simulink model "ibvs_lite_model"  (R2020b)
settings: Solver=ode45  StartTime=0.0  StopTime=inf  RelTol=1e-3  EnableMultiTasking=on
values from neighbouring files (symbols this model uses):
  q0 = zeros(7,1)    [setup.m]
  x0 = [T.t', tr2rpy(T)]    [setup.m]
undefined symbols (not defined in the file or in its folder): cond, LWR, mkgrid, nofriction, transl, troty, trotz
libraries: roblocks x19, simulink x4
(part 1 of 2)
settings Model: Creator=corkep  LastModifiedBy=kika
settings SolverCC: AlgebraicLoopSolver=LineSearch
settings DataIOCC: LimitDataPoints=on  SaveFormat=Array  TimeSaveName=t  OutputSaveName=y  ReturnWorkspaceOutputsName=opspace
settings OptimizationCC: LifeSpan=inf
settings DebuggingCC: AllowSymbolicDim=off  SFUnexpectedBacktrackingDiag=warning  SFNoUnconditionalDefaultTransitionDiag=warning  SFExecutionAtInitializationDiag=none  ArithmeticOperatorsInVariantConditions=warning
settings ModelReferenceCC: PropagateSignalLabelsOutOfModel=off
settings SFSimCC: SimUseLocalCustomCode=off  CustomCodeUndefinedFunction=UseInterfaceOnly
settings RTWCC: RTWUseLocalCustomCode=off
settings CodeAppCC: StateflowObjectComments=on
settings GRTTargetCC: TargetLangStandard=C89/C90 (ANSI)
settings ConfigComp: CovMetricSettings=dw  CovSaveCumulativeToWorkspaceVar=on  CovSaveSingleToWorkspaceVar=on  CovExternalEMLEnable=off

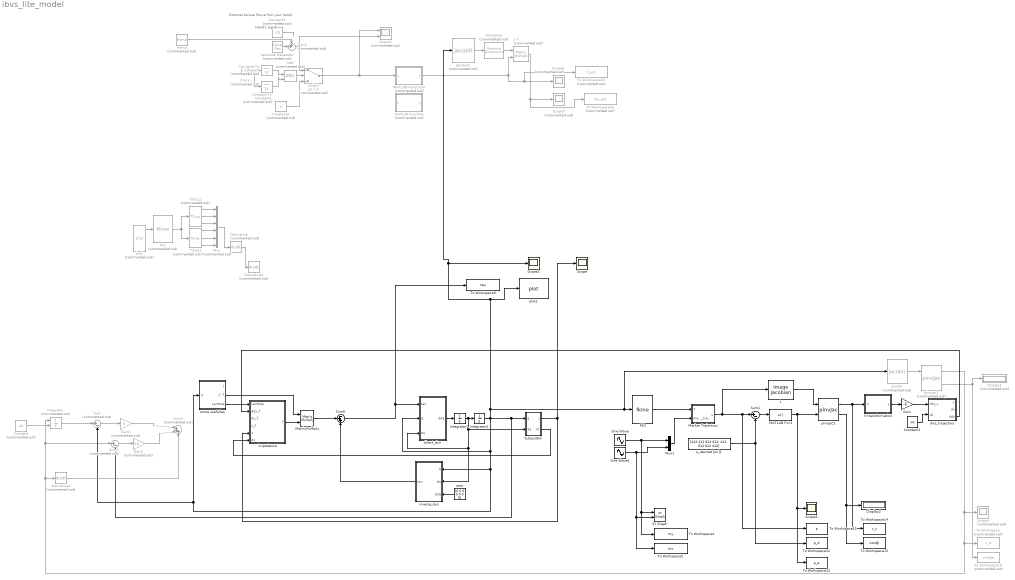
== system ibvs_lite_model ==
  note: Hand's signal
  note: External torque (force fron your hand)
  AND : Logic  Commented=on  IconShape=distinctive  AllPortsSameDT=off  OutDataTypeStr=boolean
  Clock : Clock  Commented=on
  Compare To Constant : simulink/Logic and Bit Operations/Compare To Constant  Commented=on  relop=>=  const=10  OutDataTypeStr=boolean
  Compare To Constant1 : simulink/Logic and Bit Operations/Compare To Constant  Commented=on  relop=<=  const=15  OutDataTypeStr=boolean
  Constant : Constant  Commented=on  Value=q0
  Constant1 : Constant  Value=x0
  Constant3 : Constant  Commented=on  Value=0
  Constant4 : Constant  Commented=on  Value=-25
  Derivative : Derivative  Commented=on
  Derivative1 : Derivative  Commented=on
  Derivative2 : Derivative  Commented=on
  Display1 : Display  Commented=on
  Display2 : Display
  FK1 : roblocks/Arm/fkine  Commented=on  robot=LWR
  FK2 : roblocks/Arm/fkine  robot=nofriction(LWR)
  Gain : Gain  Gain=-6
  Gain1 : Gain  Commented=on  Gain=5
  Gain2 : Gain  Commented=on  Gain=10
  Integrator : Integrator  Commented=on  InitialConditionSource=external  InitialCondition=q0'
  Integrator1 : Integrator
  Integrator2 : Integrator  InitialCondition=q0
  J' F : Product  Commented=on  Multiplication=Matrix(*)
  Jacobian : roblocks/Arm/jacob0   Commented=on  robot=LWR
  L : roblocks/Vision/image Jacobian  cam=cam  z=1
  MATLAB Fcn1 : MATLABFcn  MATLABFcn=u(:)  Output1D=off
  MATLAB Function : MATLAB Function  Commented=on  TreatAsAtomicUnit=on
  MATLAB Function3 : MATLAB Function  Commented=on  TreatAsAtomicUnit=on
  Marker Trajectory : Subsystem
  MatrixMultiply : Product  Multiplication=Matrix(*)
  Mux : Mux  Commented=on  Inputs=6
  Mux1 : Mux  Inputs=2
  Ramp : simulink/Sources/Ramp  Commented=on  slope=1  start=10  InitialOutput=-25
  Sawtooth Generator : SignalGenerator  Commented=on  Amplitude=18  Frequency=0.1  Units=rad/sec
  Scope : Scope
  Scope1 : Scope  Commented=on
  Scope2 : Scope
  Scope3 : Scope  Commented=on  NumInputPorts=2
  Scope4 : Scope
  Scope5 : Scope  Commented=on
  Scope6 : Scope  Commented=on
  Sine Wave : Sin  Amplitude=0.3  Frequency=0.3  SampleTime=0
  Sine Wave1 : Sin  Amplitude=0.3  Frequency=0.3  Phase=pi/2  SampleTime=0
  Subsystem : Subsystem
  Sum : Sum  Commented=on  Inputs=|+-
  Sum1 : Sum  Inputs=|+-
  Sum2 : Sum  Commented=on  Inputs=|+-
  Sum3 : Sum  Commented=on  Inputs=++|
  Sum4 : Sum  Commented=on  Inputs=|+++
  Sum6 : Sum  Inputs=-++  InputSameDT=on  SaturateOnIntegerOverflow=on  OutDataTypeStr=Inherit: Same as first input
  Switch : Switch  Commented=on  Criteria=u2 > Threshold
  T2rpy1 : roblocks/Toolbox/T2rpy  Commented=on  sequence=ZYX  degrees=off
  T2xyz1 : roblocks/Toolbox/T2xyz  Commented=on
  To Workspace : ToWorkspace  Commented=on  VariableName=v_e  SaveFormat=Timeseries  SampleTime=-1
  To Workspace10 : ToWorkspace  Commented=on  VariableName=f_ext  SaveFormat=Timeseries  SampleTime=-1
  To Workspace11 : ToWorkspace  VariableName=p  SaveFormat=Timeseries  SampleTime=-1
  To Workspace12 : ToWorkspace  VariableName=p_d  SaveFormat=Timeseries  SampleTime=-1
  To Workspace13 : ToWorkspace  VariableName=p_e  SaveFormat=Timeseries  SampleTime=-1
  To Workspace14 : ToWorkspace  VariableName=v_c  SaveFormat=Timeseries  SampleTime=-1
  To Workspace15 : ToWorkspace  VariableName=condJi  SaveFormat=Timeseries  SampleTime=-1
  To Workspace16 : ToWorkspace  Commented=on  VariableName=tau_ext  SaveFormat=Timeseries  SampleTime=-1
  To Workspace19 : ToWorkspace  Commented=on  VariableName=condJe  SaveFormat=Timeseries  SampleTime=-1
  To Workspace4 : ToWorkspace  VariableName=my  SaveFormat=Timeseries  SampleTime=-1
  To Workspace5 : ToWorkspace  VariableName=mz  SaveFormat=Timeseries  SampleTime=-1
  To Workspace9 : ToWorkspace  VariableName=tau  SaveFormat=Timeseries  SampleTime=-1
  V transformation : MATLAB Function  TreatAsAtomicUnit=on
  XY Graph : simulink/Sinks/XY Graph  xmin=-1  xmax=1  ymin=-1  ymax=1  st=-1
  "direct_dyn " : MATLAB Function  TreatAsAtomicUnit=on
  ibvs_trajectory : Subsystem
  impedance : MATLAB Function  TreatAsAtomicUnit=on
  inverse_dyn : MATLAB Function  TreatAsAtomicUnit=on
  jacobn : roblocks/Arm/jacobn  Commented=on  robot=nofriction(LWR)
  jtraj : roblocks/Toolbox/jtraj  Commented=on  q0=[0 0 0 0 0 0 0]  qf=[pi/4 pi/2 -pi/2 0 pi/3 0 pi]  tmax=10  ts=0.02
  p_desired [px]1 : Constant  Value=[412 412 612 612; 412 612 612 412]  VectorParams1D=off
  pinvJac1 : roblocks/Toolbox/pinvJac  Commented=on
  pinvJac2 : roblocks/Toolbox/pinvJac
  plot1 : roblocks/Arm/plot  robot=nofriction(LWR)  fps=-1  holdplot=on
  some usefulles : Subsystem
  transpose : PermuteDimensions  Commented=on
  zero : Constant  Value=[0 0 0 0 0 0 0]
  wires:
  inverse_dyn/1(tau) -> Sum6/3
  Sum6/1 -> "direct_dyn "/1(tau), To Workspace9/1
  Jacobian/1 -> transpose/1
  transpose/1 -> J' F/1
  Constant4/1 -> ?
  Sawtooth Generator/1 -> Sum3/2
  Compare To Constant1/1 -> AND/2
  Switch/1 -> Scope3/1, MATLAB Function3/1(u)
  AND/1 -> Switch/2
  Sum3/1 -> Scope3/2, Switch/1
  Constant3/1 -> Switch/3
  Compare To Constant/1 -> AND/1
  Clock/1 -> Compare To Constant1/1, Compare To Constant/1
  MATLAB Function3/1(y) -> J' F/2, To Workspace10/1, Scope6/1
  Ramp/1 -> Sum3/1
  J' F/1 -> Scope5/1, To Workspace16/1
  Gain/1 -> ibvs_trajectory/1(dot_x)
  impedance/1(f) -> MatrixMultiply/2
  MatrixMultiply/1 -> Sum6/2
  some usefulles/2(J^T) -> MatrixMultiply/1
  some usefulles/3("Lambda ") -> impedance/1(Lambda)
  Subsystem/2(dx) -> impedance/6(dx)
  Subsystem/1(x) -> impedance/5(x), Scope/1
  jtraj/1 -> FK1/1
  FK1/1 -> T2rpy1/1, T2xyz1/1
  T2xyz1/1 -> Mux/1
  T2xyz1/2 -> Mux/2
  T2xyz1/3 -> Mux/3
  T2rpy1/1 -> Mux/4
  T2rpy1/2 -> Mux/5
  T2rpy1/3 -> Mux/6
  Mux/1 -> Derivative/1
  Derivative/1 -> Derivative1/1
  pinvJac2/2 -> To Workspace15/1, Display2/1
  FK2/1 -> Marker Trajectory/1(T)
  jacobn/1 -> pinvJac1/1
  L/1 -> pinvJac2/1
  Marker Trajectory/1(s) -> L/1, To Workspace11/1, Sum1/1
  V transformation/1(y) -> Gain/1
  MATLAB Fcn1/1 -> pinvJac2/2, To Workspace13/1, Scope4/1
  Sum1/1 -> MATLAB Fcn1/1
  pinvJac2/1 -> V transformation/1(u), To Workspace14/1
  pinvJac1/2 -> Display1/1, To Workspace19/1
  p_desired [px]1/1 -> Sum1/2, To Workspace12/1
  pinvJac1/1 -> Derivative2/1, Sum2/1, Integrator/1, To Workspace/1, Scope1/1
  Sine Wave1/1 -> XY Graph/2, To Workspace5/1, Mux1/2
  Sine Wave/1 -> To Workspace4/1, XY Graph/1, Mux1/1
  Mux1/1 -> Marker Trajectory/2("marker_traj ")
  ibvs_trajectory/3(ddx) -> impedance/2(ddx_f)
  Sum2/1 -> Gain2/1
  Sum/1 -> Gain1/1
  Gain1/1 -> Sum4/1
  Gain2/1 -> Sum4/2
  Integrator2/1 -> Sum/2, some usefulles/1(q), inverse_dyn/1(q), "direct_dyn "/2(q), Jacobian/1, Scope2/1, plot1/1, jacobn/1, FK2/1, Subsystem/1(q), Sum2/2
  Integrator/1 -> Sum/1
  Constant/1 -> Integrator/2
  Derivative2/1 -> Sum4/3
  Constant1/1 -> ibvs_trajectory/2(x0)
  Integrator1/1 -> Subsystem/2(dq), inverse_dyn/2(dq), "direct_dyn "/3(dq), Integrator2/1
  "direct_dyn "/1(ddq) -> Integrator1/1
  zero/1 -> inverse_dyn/3(ddq)

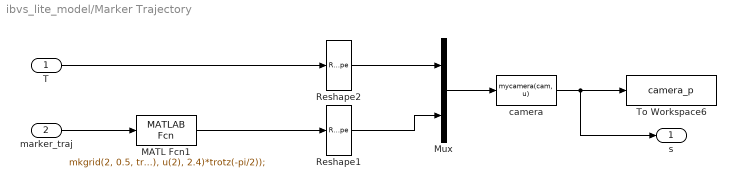
== system ibvs_lite_model/Marker Trajectory ==
  T : Inport
  "marker_traj " : Inport  Port=2
  MATL Fcn1 : MATLABFcn  MATLABFcn=mkgrid(2, 0.5, troty(pi/2)*transl(u(1), u(2), 2.4)*trotz(-pi/2));  OutputSignalType=real  Output1D=off
  Mux : Mux  Inputs=2
  Reshape1 : Reshape  OutputDimensionality=Column vector (2-D)  OutputDimensions=6
  Reshape2 : Reshape  OutputDimensionality=Column vector (2-D)  OutputDimensions=6
  To Workspace6 : ToWorkspace  VariableName=camera_p  SaveFormat=Timeseries  SampleTime=-1
  camera : MATLABFcn  MATLABFcn=mycamera(cam, u)  OutputSignalType=real  Output1D=off
  s : Outport  VectorParamsAs1DForOutWhenUnconnected=off
  wires:
  Reshape1/1 -> Mux/2
  Reshape2/1 -> Mux/1
  T/1 -> Reshape2/1
  Mux/1 -> camera/1
  camera/1 -> s/1, To Workspace6/1
  MATL Fcn1/1 -> Reshape1/1
  "marker_traj "/1 -> MATL Fcn1/1

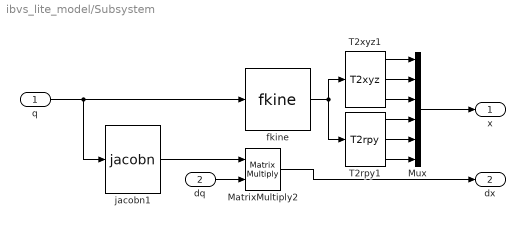
== system ibvs_lite_model/Subsystem ==
  q : Inport
  dq : Inport  Port=2
  MatrixMultiply2 : Product  Multiplication=Matrix(*)
  Mux : Mux  Inputs=6
  T2rpy1 : roblocks/Toolbox/T2rpy  sequence=ZYX  degrees=off
  T2xyz1 : roblocks/Toolbox/T2xyz
  fkine : roblocks/Arm/fkine  robot=nofriction(LWR)
  jacobn1 : roblocks/Arm/jacobn  robot=nofriction(LWR)
  x : Outport  VectorParamsAs1DForOutWhenUnconnected=off
  dx : Outport  Port=2  VectorParamsAs1DForOutWhenUnconnected=off
  wires:
  MatrixMultiply2/1 -> dx/1
  T2rpy1/3 -> Mux/6
  T2xyz1/1 -> Mux/1
  dq/1 -> MatrixMultiply2/2
  q/1 -> jacobn1/1, fkine/1
  fkine/1 -> T2rpy1/1, T2xyz1/1
  T2rpy1/2 -> Mux/5
  jacobn1/1 -> MatrixMultiply2/1
  Mux/1 -> x/1
  T2rpy1/1 -> Mux/4
  T2xyz1/2 -> Mux/2
  T2xyz1/3 -> Mux/3

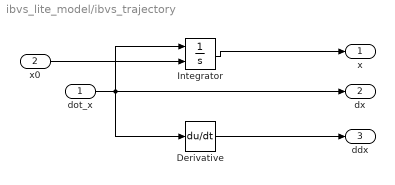
== system ibvs_lite_model/ibvs_trajectory ==
  dot_x : Inport
  x0 : Inport  Port=2
  Derivative : Derivative
  Integrator : Integrator  InitialConditionSource=external  InitialCondition=q0'
  x : Outport  VectorParamsAs1DForOutWhenUnconnected=off
  dx : Outport  Port=2  VectorParamsAs1DForOutWhenUnconnected=off
  ddx : Outport  Port=3  VectorParamsAs1DForOutWhenUnconnected=off
  wires:
  Derivative/1 -> ddx/1
  Integrator/1 -> x/1
  dot_x/1 -> Integrator/1, dx/1, Derivative/1
  x0/1 -> Integrator/2

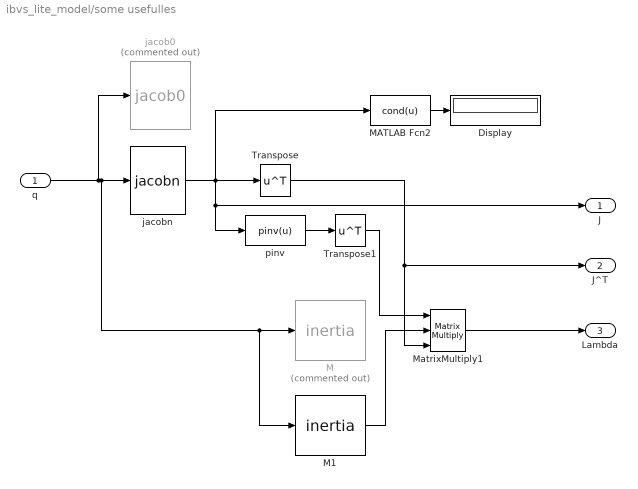
== system ibvs_lite_model/some usefulles ==
  q : Inport
  Display : Display
  M : roblocks/Arm/inertia  Commented=on  robot=nofriction(LWR)
  M1 : roblocks/Arm/inertia  robot=nofriction(LWR)
  MATLAB Fcn2 : MATLABFcn  MATLABFcn=cond(u)  Output1D=off
  MatrixMultiply1 : Product  Inputs=3  Multiplication=Matrix(*)
  Transpose : Math  Operator=transpose  SignedPower=on  SaturateOnIntegerOverflow=on
  Transpose1 : Math  Operator=transpose  SignedPower=on  SaturateOnIntegerOverflow=on
  "jacob0 " : roblocks/Arm/jacob0   Commented=on  robot=nofriction(LWR)
  jacobn : roblocks/Arm/jacobn  robot=nofriction(LWR)
  pinv : MATLABFcn  MATLABFcn=pinv(u)  Output1D=off
  J : Outport  VectorParamsAs1DForOutWhenUnconnected=off
  J^T : Outport  Port=2  VectorParamsAs1DForOutWhenUnconnected=off
  "Lambda " : Outport  Port=3  VectorParamsAs1DForOutWhenUnconnected=off
  wires:
  pinv/1 -> Transpose1/1
  q/1 -> "jacob0 "/1, M1/1, M/1, jacobn/1
  M1/1 -> MatrixMultiply1/2
  Transpose1/1 -> MatrixMultiply1/1
  MatrixMultiply1/1 -> "Lambda "/1
  jacobn/1 -> MATLAB Fcn2/1, J/1, pinv/1, Transpose/1
  Transpose/1 -> J^T/1, MatrixMultiply1/3
  MATLAB Fcn2/1 -> Display/1

== matlab function ibvs_lite_model/MATLAB Function ==
  data: u input; y output
function y = fcn(u)

y = [u, 0, 0, 0, 0, 0, 0];

== matlab function ibvs_lite_model/V transformation ==
  data: u input; y output
function y = fcn(u)
R = [
        -1         0         0;
         0         1         0;
         0         0        -1
];

V = [
    R,  zeros(3,3);
    zeros(3,3), R
];

% u = V * u;
y = u;

== matlab function ibvs_lite_model/direct_dyn  ==
  data: tau input; ddq output size=7; q input; dq input
function ddq = ddm(tau, q, dq)

q1 = q(1);
q2 = q(2);
q3 = q(3);
q4 = q(4);
q5 = q(5);
q6 = q(6);
q7 = q(7);

QP1 = dq(1);
QP2 = dq(2);
QP3 = dq(3);
QP4 = dq(4);
QP5 = dq(5);
QP6 = dq(6);
QP7 = dq(7);

GAM1 = tau(1);
GAM2 = tau(2);
GAM3 = tau(3);
GAM4 = tau(4);
GAM5 = tau(5);
GAM6 = tau(6);
GAM7 = tau(7);


radius = 0.05;

l1 = 0.1;
M1 = 2;

XX1 = 1/12 * M1 * l1 * l1;
XY1 = 0;
XZ1 = 0;
YY1 = 1/12 * M1 * l1 * l1;
YZ1 = 0;
ZZ1 = 1/2 * M1 * radius;
MX1 = 0;
MY1 = 0;
MZ1 = M1 * l1;

l2 = 0.1;
M2 = 2;

XX2 = 1/12 * M2 * l2 * l2;
XY2 = 0;
XZ2 = 0;
YY2 = 1/2 * M2 * radius;
YZ2 = 0;
ZZ2 = 1/12 * M2 * l2 * l2;
MX2 = 0;
MY2 = -M2 * l2;
MZ2 = 0;

l3 = 0.1;
M3 = 1.5;

XX3 = 1/12 * M3 * l3 * l3;
XY3 = 0;
XZ3 = 0;
YY3 = 1/12 * M3 * l3 * l3;
YZ3 = 0;
ZZ3 = 1/2 * M3 * radius;
MX3 = 0;
MY3 = 0;
MZ3 = M3 * l3;

l4 = 0.1;
M4 = 1.5;

XX4 = 1/12 * M4 * l4 * l4;
XY4 = 0;
XZ4 = 0;
YY4 = 1/2 * M4 * radius;
YZ4 = 0;
ZZ4 = 1/12 * M4 * l4 * l4;
MX4 = 0;
MY4 = M4 * 0.1;
MZ4 = 0;

l5 = 0.1;
M5 = 1.5;

XX5 = 1/12 * M5 * l5 * l5;
XY5 = 0;
XZ5 = 0;
YY5 = 1/12 * M5 * l5 * l5;
YZ5 = 0;
ZZ5 = 1/2 * M5 * radius;
MX5 = 0;
MY5 = 0;
MZ5 = M5 * l5;

l6 = 0.1;
M6 = 1;

XX6 = 1/12 * M6 * l6 * l6;
XY6 = 0;
XZ6 = 0;
YY6 = 1/12 * M6 * l6 * l6;
YZ6 = 0;
ZZ6 = 1/2 * M6 * radius;
MX6 = 0;
MY6 = -M6 * l6;
MZ6 = 0;

l7 = 0.05;
M7 = 0.1;

XX7 = 1/12 * M7 * l7 * l7;
XY7 = 0;
XZ7 = 0;
YY7 = 1/12 * M7 * l7 * l7;
YZ7 = 0;
ZZ7 = 1/2 * M7 * radius;
MX7 = 0;
MY7 = 0;
MZ7 = M7 * l7;


FX7 = 0;
FY7 = 0;
FZ7 = 0;
CX7 = 0;
CY7 = 0;
CZ7 = 0;


C1 = cos(q1);
S1 = sin(q1);
C2 = cos(q2);
S2 = sin(q2);
C3 = cos(q3);
S3 = sin(q3);
C4 = cos(q4);
S4 = sin(q4);
C5 = cos(q5);
S5 = sin(q5);
C6 = cos(q6);
S6 = sin(q6);
C7 = cos(q7);
S7 = sin(q7);
JW11 = QP1*XZ1;
JW21 = QP1*YZ1;
JW31 = QP1*ZZ1;
KW11 = -JW21*QP1;
KW21 = JW11*QP1;
SW11 = -MX1*QP1^2;
SW21 = -MY1*QP1^2;
WI12 = QP1*S2;
WI22 = C2*QP1;
WQ12 = QP2*WI22;
WQ22 = -QP2*WI12;
JW12 = QP2*XZ2 + WI12*XX2 + WI22*XY2;
JW22 = QP2*YZ2 + WI12*XY2 + WI22*YY2;
JW32 = QP2*ZZ2 + WI12*XZ2 + WI22*YZ2;
KW12 = -JW22*QP2 + JW32*WI22;
KW22 = JW12*QP2 - JW32*WI12;
KW32 = -JW12*WI22 + JW22*WI12;
SW12 = -QP2*(MX2*QP2 - MZ2*WI12) + WI22*(-MX2*WI22 + MY2*WI12);
SW22 = QP2*(-MY2*QP2 + MZ2*WI22) - WI12*(-MX2*WI22 + MY2*WI12);
SW32 = WI12*(MX2*QP2 - MZ2*WI12) - WI22*(-MY2*QP2 + MZ2*WI22);
WI13 = C3*WI12 - QP2*S3;
WI23 = -C3*QP2 - S3*WI12;
W33 = QP3 + WI22;
JPR123 = 0.4*S3;
JPR223 = 0.4*C3;
WQ13 = QP3*WI23;
WQ23 = -QP3*WI13;
LW13 = C3*(-0.4*QP2^2 - 0.4*WI22^2) - 0.4*QP2*S3*WI12;
LW23 = -0.4*C3*QP2*WI12 - S3*(-0.4*QP2^2 - 0.4*WI22^2);
LW33 = 0.4*WI12*WI22;
JW13 = W33*XZ3 + WI13*XX3 + WI23*XY3;
JW23 = W33*YZ3 + WI13*XY3 + WI23*YY3;
JW33 = W33*ZZ3 + WI13*XZ3 + WI23*YZ3;
KW13 = -JW23*W33 + JW33*WI23;
KW23 = JW13*W33 - JW33*WI13;
KW33 = -JW13*WI23 + JW23*WI13;
SW13 = -W33*(MX3*W33 - MZ3*WI13) + WI23*(-MX3*WI23 + MY3*WI13);
SW23 = W33*(-MY3*W33 + MZ3*WI23) - WI13*(-MX3*WI23 + MY3*WI13);
SW33 = WI13*(MX3*W33 - MZ3*WI13) - WI23*(-MY3*W33 + MZ3*WI23);
WI14 = C4*WI13 - S4*W33;
WI24 = -C4*W33 - S4*WI13;
W34 = QP4 + WI23;
WQ14 = QP4*WI24;
WQ24 = -QP4*WI14;
JW14 = W34*XZ4 + WI14*XX4 + WI24*XY4;
JW24 = W34*YZ4 + WI14*XY4 + WI24*YY4;
JW34 = W34*ZZ4 + WI14*XZ4 + WI24*YZ4;
KW14 = -JW24*W34 + JW34*WI24;
KW24 = JW14*W34 - JW34*WI14;
KW34 = -JW14*WI24 + JW24*WI14;
SW14 = -W34*(MX4*W34 - MZ4*WI14) + WI24*(-MX4*WI24 + MY4*WI14);
SW24 = W34*(-MY4*W34 + MZ4*WI24) - WI14*(-MX4*WI24 + MY4*WI14);
SW34 = WI14*(MX4*W34 - MZ4*WI14) - WI24*(-MY4*W34 + MZ4*WI24);
WI15 = C5*WI14 + S5*W34;
WI25 = C5*W34 - S5*WI14;
W35 = QP5 - WI24;
JPR125 = -0.39*S5;
JPR225 = -0.39*C5;
WQ15 = QP5*WI25;
WQ25 = -QP5*WI15;
LW15 = C5*(-0.39*W34^2 - 0.39*WI24^2) + 0.39*S5*W34*WI14;
LW25 = 0.39*C5*W34*WI14 - S5*(-0.39*W34^2 - 0.39*WI24^2);
LW35 = -0.39*WI14*WI24;
JW15 = W35*XZ5 + WI15*XX5 + WI25*XY5;
JW25 = W35*YZ5 + WI15*XY5 + WI25*YY5;
JW35 = W35*ZZ5 + WI15*XZ5 + WI25*YZ5;
KW15 = -JW25*W35 + JW35*WI25;
KW25 = JW15*W35 - JW35*WI15;
KW35 = -JW15*WI25 + JW25*WI15;
SW15 = -W35*(MX5*W35 - MZ5*WI15) + WI25*(-MX5*WI25 + MY5*WI15);
SW25 = W35*(-MY5*W35 + MZ5*WI25) - WI15*(-MX5*WI25 + MY5*WI15);
SW35 = WI15*(MX5*W35 - MZ5*WI15) - WI25*(-MY5*W35 + MZ5*WI25);
WI16 = C6*WI15 + S6*W35;
WI26 = C6*W35 - S6*WI15;
W36 = QP6 - WI25;
WQ16 = QP6*WI26;
WQ26 = -QP6*WI16;
JW16 = W36*XZ6 + WI16*XX6 + WI26*XY6;
JW26 = W36*YZ6 + WI16*XY6 + WI26*YY6;
JW36 = W36*ZZ6 + WI16*XZ6 + WI26*YZ6;
KW16 = -JW26*W36 + JW36*WI26;
KW26 = JW16*W36 - JW36*WI16;
KW36 = -JW16*WI26 + JW26*WI16;
SW16 = -W36*(MX6*W36 - MZ6*WI16) + WI26*(-MX6*WI26 + MY6*WI16);
SW26 = W36*(-MY6*W36 + MZ6*WI26) - WI16*(-MX6*WI26 + MY6*WI16);
SW36 = WI16*(MX6*W36 - MZ6*WI16) - WI26*(-MY6*W36 + MZ6*WI26);
WI17 = C7*WI16 - S7*W36;
WI27 = -C7*W36 - S7*WI16;
W37 = QP7 + WI26;
WQ17 = QP7*WI27;
WQ27 = -QP7*WI17;
JW17 = W37*XZ7 + WI17*XX7 + WI27*XY7;
JW27 = W37*YZ7 + WI17*XY7 + WI27*YY7;
JW37 = W37*ZZ7 + WI17*XZ7 + WI27*YZ7;
KW17 = -JW27*W37 + JW37*WI27;
KW27 = JW17*W37 - JW37*WI17;
KW37 = -JW17*WI27 + JW27*WI17;
SW17 = -W37*(MX7*W37 - MZ7*WI17) + WI27*(-MX7*WI27 + MY7*WI17);
SW27 = W37*(-MY7*W37 + MZ7*WI27) - WI17*(-MX7*WI27 + MY7*WI17);
SW37 = WI17*(MX7*W37 - MZ7*WI17) - WI27*(-MY7*W37 + MZ7*WI27);
BETA17 = -FX7 - SW17;
BETA27 = -FY7 - SW27;
BETA37 = -FZ7 - SW37;
BETA47 = -CX7 - KW17;
BETA57 = -CY7 - KW27;
BETA67 = -CZ7 - KW37;
GW7 = BETA67 + GAM7;
JD7 = 1/ZZ7;
JU17 = -JD7*MY7;
JU27 = JD7*MX7;
JU47 = JD7*XZ7;
JU57 = JD7*YZ7;
JU67 = JD7*ZZ7;
GK117 = JU17*MY7 + M7;
GK217 = JU27*MY7;
GK417 = JU47*MY7;
GK517 = JU57*MY7 + MZ7;
GK617 = JU67*MY7 - MY7;
GK127 = -JU17*MX7;
GK227 = -JU27*MX7 + M7;
GK427 = -JU47*MX7 - MZ7;
GK527 = -JU57*MX7;
GK627 = -JU67*MX7 + MX7;
GK147 = -JU17*XZ7;
GK247 = -JU27*XZ7 - MZ7;
GK447 = -JU47*XZ7 + XX7;
GK547 = -JU57*XZ7 + XY7;
GK647 = -JU67*XZ7 + XZ7;
GK157 = -JU17*YZ7 + MZ7;
GK257 = -JU27*YZ7;
GK457 = -JU47*YZ7 + XY7;
GK557 = -JU57*YZ7 + YY7;
GK657 = -JU67*YZ7 + YZ7;
GK167 = -JU17*ZZ7 - MY7;
GK267 = -JU27*ZZ7 + MX7;
GK467 = -JU47*ZZ7 + XZ7;
GK567 = -JU57*ZZ7 + YZ7;
GK667 = -JU67*ZZ7 + ZZ7;
NG17 = GK147*WQ17 + GK157*WQ27;
NG27 = GK247*WQ17 + GK257*WQ27;
NG37 = -MX7*WQ27 + MY7*WQ17;
NG47 = GK447*WQ17 + GK457*WQ27;
NG57 = GK547*WQ17 + GK557*WQ27;
NG67 = GK647*WQ17 + GK657*WQ27;
VS17 = GW7*JU17 + NG17;
VS27 = GW7*JU27 + NG27;
VS47 = GW7*JU47 + NG47;
VS57 = GW7*JU57 + NG57;
VS67 = GW7*JU67 + NG67;
AP17 = -BETA17 + VS17;
AP27 = -BETA27 + VS27;
AP37 = -BETA37 + NG37;
AP47 = -BETA47 + VS47;
AP57 = -BETA57 + VS57;
AP67 = -BETA67 + VS67;
GX117 = C7*GK117 - GK217*S7;
GX317 = -C7*GK217 - GK117*S7;
GX417 = C7*GK417 - GK517*S7;
GX617 = -C7*GK517 - GK417*S7;
GX127 = C7*GK127 - GK227*S7;
GX327 = -C7*GK227 - GK127*S7;
GX427 = C7*GK427 - GK527*S7;
GX627 = -C7*GK527 - GK427*S7;
GX437 = C7*MY7 + MX7*S7;
GX637 = C7*MX7 - MY7*S7;
GX147 = C7*GK147 - GK247*S7;
GX347 = -C7*GK247 - GK147*S7;
GX447 = C7*GK447 - GK547*S7;
GX647 = -C7*GK547 - GK447*S7;
GX157 = C7*GK157 - GK257*S7;
GX357 = -C7*GK257 - GK157*S7;
GX457 = C7*GK457 - GK557*S7;
GX657 = -C7*GK557 - GK457*S7;
GX167 = C7*GK167 - GK267*S7;
GX367 = -C7*GK267 - GK167*S7;
GX467 = C7*GK467 - GK567*S7;
GX667 = -C7*GK567 - GK467*S7;
TKT117 = C7*GX117 - GX127*S7;
TKT317 = C7*GX317 - GX327*S7;
TKT417 = C7*GX417 - GX427*S7;
TKT517 = C7*GK617 - GK627*S7;
TKT617 = C7*GX617 - GX627*S7;
TKT337 = -C7*GX327 - GX317*S7;
TKT437 = -C7*GX427 - GX417*S7;
TKT537 = -C7*GK627 - GK617*S7;
TKT637 = -C7*GX627 - GX617*S7;
TKT447 = C7*GX447 - GX457*S7;
TKT547 = C7*GK647 - GK657*S7;
TKT647 = C7*GX647 - GX657*S7;
TKT667 = -C7*GX657 - GX647*S7;
ALJI17 = AP17*C7 - AP27*S7;
ALJI37 = -AP17*S7 - AP27*C7;
ALJI47 = AP47*C7 - AP57*S7;
ALJI67 = -AP47*S7 - AP57*C7;
MJE116 = M6 + TKT117;
MJE516 = MZ6 + TKT517;
MJE616 = -MY6 + TKT617;
MJE226 = M6 + M7;
MJE426 = GX437 - MZ6;
MJE626 = GX637 + MX6;
MJE336 = M6 + TKT337;
MJE436 = MY6 + TKT437;
MJE536 = -MX6 + TKT537;
MJE446 = TKT447 + XX6;
MJE546 = TKT547 + XY6;
MJE646 = TKT647 + XZ6;
MJE556 = GK667 + YY6;
MJE656 = GX667 + YZ6;
MJE666 = TKT667 + ZZ6;
VBE16 = -ALJI17 - SW16;
VBE26 = -AP37 - SW26;
VBE36 = -ALJI37 - SW36;
VBE46 = -ALJI47 - KW16;
VBE56 = -AP67 - KW26;
VBE66 = -ALJI67 - KW36;
GW6 = GAM6 + VBE66;
JD6 = 1/MJE666;
JU16 = JD6*MJE616;
JU26 = JD6*MJE626;
JU36 = JD6*TKT637;
JU46 = JD6*MJE646;
JU56 = JD6*MJE656;
JU66 = JD6*MJE666;
GK116 = -JU16*MJE616 + MJE116;
GK216 = -JU26*MJE616;
GK316 = -JU36*MJE616 + TKT317;
GK416 = -JU46*MJE616 + TKT417;
GK516 = -JU56*MJE616 + MJE516;
GK616 = -JU66*MJE616 + MJE616;
GK126 = -JU16*MJE626;
GK226 = -JU26*MJE626 + MJE226;
GK326 = -JU36*MJE626;
GK426 = -JU46*MJE626 + MJE426;
GK526 = -JU56*MJE626;
GK626 = -JU66*MJE626 + MJE626;
GK136 = -JU16*TKT637 + TKT317;
GK236 = -JU26*TKT637;
GK336 = -JU36*TKT637 + MJE336;
GK436 = -JU46*TKT637 + MJE436;
GK536 = -JU56*TKT637 + MJE536;
GK636 = -JU66*TKT637 + TKT637;
GK146 = -JU16*MJE646 + TKT417;
GK246 = -JU26*MJE646 + MJE426;
GK346 = -JU36*MJE646 + MJE436;
GK446 = -JU46*MJE646 + MJE446;
GK546 = -JU56*MJE646 + MJE546;
GK646 = -JU66*MJE646 + MJE646;
GK156 = -JU16*MJE656 + MJE516;
GK256 = -JU26*MJE656;
GK356 = -JU36*MJE656 + MJE536;
GK456 = -JU46*MJE656 + MJE546;
GK556 = -JU56*MJE656 + MJE556;
GK656 = -JU66*MJE656 + MJE656;
GK166 = -JU16*MJE666 + MJE616;
GK266 = -JU26*MJE666 + MJE626;
GK366 = -JU36*MJE666 + TKT637;
GK466 = -JU46*MJE666 + MJE646;
GK566 = -JU56*MJE666 + MJE656;
GK666 = -JU66*MJE666 + MJE666;
NG16 = GK146*WQ16 + GK156*WQ26;
NG26 = GK246*WQ16 + GK256*WQ26;
NG36 = GK346*WQ16 + GK356*WQ26;
NG46 = GK446*WQ16 + GK456*WQ26;
NG56 = GK546*WQ16 + GK556*WQ26;
NG66 = GK646*WQ16 + GK656*WQ26;
VS16 = GW6*JU16 + NG16;
VS26 = GW6*JU26 + NG26;
VS36 = GW6*JU36 + NG36;
VS46 = GW6*JU46 + NG46;
VS56 = GW6*JU56 + NG56;
VS66 = GW6*JU66 + NG66;
AP16 = -VBE16 + VS16;
AP26 = -VBE26 + VS26;
AP36 = -VBE36 + VS36;
AP46 = -VBE46 + VS46;
AP56 = -VBE56 + VS56;
AP66 = -VBE66 + VS66;
GX116 = C6*GK116 - GK216*S6;
GX316 = C6*GK216 + GK116*S6;
GX416 = C6*GK416 - GK516*S6;
GX616 = C6*GK516 + GK416*S6;
GX126 = C6*GK126 - GK226*S6;
GX326 = C6*GK226 + GK126*S6;
GX426 = C6*GK426 - GK526*S6;
GX626 = C6*GK526 + GK426*S6;
GX136 = C6*GK136 - GK236*S6;
GX336 = C6*GK236 + GK136*S6;
GX436 = C6*GK436 - GK536*S6;
GX636 = C6*GK536 + GK436*S6;
GX146 = C6*GK146 - GK246*S6;
GX346 = C6*GK246 + GK146*S6;
GX446 = C6*GK446 - GK546*S6;
GX646 = C6*GK546 + GK446*S6;
GX156 = C6*GK156 - GK256*S6;
GX356 = C6*GK256 + GK156*S6;
GX456 = C6*GK456 - GK556*S6;
GX656 = C6*GK556 + GK456*S6;
GX166 = C6*GK166 - GK266*S6;
GX366 = C6*GK266 + GK166*S6;
GX466 = C6*GK466 - GK566*S6;
GX666 = C6*GK566 + GK466*S6;
TKT116 = C6*GX116 - GX126*S6;
TKT216 = -C6*GK316 + GK326*S6;
TKT316 = C6*GX316 - GX326*S6;
TKT416 = C6*GX416 - GX426*S6;
TKT516 = -C6*GK616 + GK626*S6;
TKT616 = C6*GX616 - GX626*S6;
TKT336 = C6*GX326 + GX316*S6;
TKT436 = C6*GX426 + GX416*S6;
TKT536 = -C6*GK626 - GK616*S6;
TKT636 = C6*GX626 + GX616*S6;
TKT446 = C6*GX446 - GX456*S6;
TKT546 = -C6*GK646 + GK656*S6;
TKT646 = C6*GX646 - GX656*S6;
TKT666 = C6*GX656 + GX646*S6;
ALJI16 = AP16*C6 - AP26*S6;
ALJI36 = AP16*S6 + AP26*C6;
ALJI46 = AP46*C6 - AP56*S6;
ALJI66 = AP46*S6 + AP56*C6;
MJE115 = M5 + TKT116;
MJE515 = MZ5 + TKT516;
MJE615 = -MY5 + TKT616;
MJE225 = GK336 + M5;
MJE425 = -GX436 - MZ5;
MJE625 = -GX636 + MX5;
MJE335 = M5 + TKT336;
MJE435 = MY5 + TKT436;
MJE535 = -MX5 + TKT536;
MJE445 = TKT446 + XX5;
MJE545 = TKT546 + XY5;
MJE645 = TKT646 + XZ5;
MJE555 = GK666 + YY5;
MJE655 = -GX666 + YZ5;
MJE665 = TKT666 + ZZ5;
VBE15 = -ALJI16 - SW15;
VBE25 = AP36 - SW25;
VBE35 = -ALJI36 - SW35;
VBE45 = -ALJI46 - KW15;
VBE55 = AP66 - KW25;
VBE65 = -ALJI66 - KW35;
GW5 = GAM5 + VBE65;
JD5 = 1/MJE665;
JU15 = JD5*MJE615;
JU25 = JD5*MJE625;
JU35 = JD5*TKT636;
JU45 = JD5*MJE645;
JU55 = JD5*MJE655;
JU65 = JD5*MJE665;
GK115 = -JU15*MJE615 + MJE115;
GK215 = -JU25*MJE615 + TKT216;
GK315 = -JU35*MJE615 + TKT316;
GK415 = -JU45*MJE615 + TKT416;
GK515 = -JU55*MJE615 + MJE515;
GK615 = -JU65*MJE615 + MJE615;
GK125 = -JU15*MJE625 + TKT216;
GK225 = -JU25*MJE625 + MJE225;
GK325 = -GX336 - JU35*MJE625;
GK425 = -JU45*MJE625 + MJE425;
GK525 = GK636 - JU55*MJE625;
GK625 = -JU65*MJE625 + MJE625;
GK135 = -JU15*TKT636 + TKT316;
GK235 = -GX336 - JU25*TKT636;
GK335 = -JU35*TKT636 + MJE335;
GK435 = -JU45*TKT636 + MJE435;
GK535 = -JU55*TKT636 + MJE535;
GK635 = -JU65*TKT636 + TKT636;
GK145 = -JU15*MJE645 + TKT416;
GK245 = -JU25*MJE645 + MJE425;
GK345 = -JU35*MJE645 + MJE435;
GK445 = -JU45*MJE645 + MJE445;
GK545 = -JU55*MJE645 + MJE545;
GK645 = -JU65*MJE645 + MJE645;
GK155 = -JU15*MJE655 + MJE515;
GK255 = GK636 - JU25*MJE655;
GK355 = -JU35*MJE655 + MJE535;
GK455 = -JU45*MJE655 + MJE545;
GK555 = -JU55*MJE655 + MJE555;
GK655 = -JU65*MJE655 + MJE655;
GK165 = -JU15*MJE665 + MJE615;
GK265 = -JU25*MJE665 + MJE625;
GK365 = -JU35*MJE665 + TKT636;
GK465 = -JU45*MJE665 + MJE645;
GK565 = -JU55*MJE665 + MJE655;
GK665 = -JU65*MJE665 + MJE665;
NG15 = GK115*LW15 + GK125*LW25 + GK135*LW35 + GK145*WQ15 + GK155*WQ25;
NG25 = GK215*LW15 + GK225*LW25 + GK235*LW35 + GK245*WQ15 + GK255*WQ25;
NG35 = GK315*LW15 + GK325*LW25 + GK335*LW35 + GK345*WQ15 + GK355*WQ25;
NG45 = GK415*LW15 + GK425*LW25 + GK435*LW35 + GK445*WQ15 + GK455*WQ25;
NG55 = GK515*LW15 + GK525*LW25 + GK535*LW35 + GK545*WQ15 + GK555*WQ25;
NG65 = GK615*LW15 + GK625*LW25 + GK635*LW35 + GK645*WQ15 + GK655*WQ25;
VS15 = GW5*JU15 + NG15;
VS25 = GW5*JU25 + NG25;
VS35 = GW5*JU35 + NG35;
VS45 = GW5*JU45 + NG45;
VS55 = GW5*JU55 + NG55;
VS65 = GW5*JU65 + NG65;
AP15 = -VBE15 + VS15;
AP25 = -VBE25 + VS25;
AP35 = -VBE35 + VS35;
AP45 = -VBE45 + VS45;
AP55 = -VBE55 + VS55;
AP65 = -VBE65 + VS65;
GX115 = C5*GK115 - GK215*S5;
GX315 = C5*GK215 + GK115*S5;
GX415 = C5*GK415 - GK515*S5;
GX515 = GK115*JPR125 + GK215*JPR225 - GK615;
GX615 = C5*GK515 - 0.39*GK315 + GK415*S5;
GX125 = C5*GK125 - GK225*S5;
GX325 = C5*GK225 + GK125*S5;
GX425 = C5*GK425 - GK525*S5;
GX525 = GK125*JPR125 + GK225*JPR225 - GK625;
GX625 = C5*GK525 - 0.39*GK325 + GK425*S5;
GX135 = C5*GK135 - GK235*S5;
GX335 = C5*GK235 + GK135*S5;
GX435 = C5*GK435 - GK535*S5;
GX535 = GK135*JPR125 + GK235*JPR225 - GK635;
GX635 = C5*GK535 - 0.39*GK335 + GK435*S5;
GX145 = C5*GK145 - GK245*S5;
GX345 = C5*GK245 + GK145*S5;
GX445 = C5*GK445 - GK545*S5;
GX545 = GK145*JPR125 + GK245*JPR225 - GK645;
GX645 = C5*GK545 - 0.39*GK345 + GK445*S5;
GX155 = C5*GK155 - GK255*S5;
GX355 = C5*GK255 + GK155*S5;
GX455 = C5*GK455 - GK555*S5;
GX555 = GK155*JPR125 + GK255*JPR225 - GK655;
GX655 = C5*GK555 - 0.39*GK355 + GK455*S5;
GX165 = C5*GK165 - GK265*S5;
GX365 = C5*GK265 + GK165*S5;
GX465 = C5*GK465 - GK565*S5;
GX565 = GK165*JPR125 + GK265*JPR225 - GK665;
GX665 = C5*GK565 - 0.39*GK365 + GK465*S5;
TKT115 = C5*GX115 - GX125*S5;
TKT215 = -C5*GK315 + GK325*S5;
TKT315 = C5*GX315 - GX325*S5;
TKT415 = C5*GX415 - GX425*S5;
TKT515 = C5*GX515 - GX525*S5;
TKT615 = C5*GX615 - GX625*S5;
TKT335 = C5*GX325 + GX315*S5;
TKT435 = C5*GX425 + GX415*S5;
TKT535 = C5*GX525 + GX515*S5;
TKT635 = C5*GX625 + GX615*S5;
TKT445 = C5*GX445 - GX455*S5;
TKT545 = C5*GX545 - GX555*S5;
TKT645 = C5*GX645 - GX655*S5;
TKT555 = GX515*JPR125 + GX525*JPR225 - GX565;
TKT655 = GX615*JPR125 + GX625*JPR225 - GX665;
TKT665 = C5*GX655 - 0.39*GX635 + GX645*S5;
ALJI15 = AP15*C5 - AP25*S5;
ALJI35 = AP15*S5 + AP25*C5;
ALJI45 = AP45*C5 - AP55*S5;
ALJI55 = AP15*JPR125 + AP25*JPR225 - AP65;
ALJI65 = -0.39*AP35 + AP45*S5 + AP55*C5;
MJE114 = M4 + TKT115;
MJE514 = MZ4 + TKT515;
MJE614 = -MY4 + TKT615;
MJE224 = GK335 + M4;
MJE424 = -GX435 - MZ4;
MJE624 = -GX635 + MX4;
MJE334 = M4 + TKT335;
MJE434 = MY4 + TKT435;
MJE534 = -MX4 + TKT535;
MJE444 = TKT445 + XX4;
MJE544 = TKT545 + XY4;
MJE644 = TKT645 + XZ4;
MJE554 = TKT555 + YY4;
MJE654 = TKT655 + YZ4;
MJE664 = TKT665 + ZZ4;
VBE14 = -ALJI15 - SW14;
VBE24 = AP35 - SW24;
VBE34 = -ALJI35 - SW34;
VBE44 = -ALJI45 - KW14;
VBE54 = -ALJI55 - KW24;
VBE64 = -ALJI65 - KW34;
GW4 = GAM4 + VBE64;
JD4 = 1/MJE664;
JU14 = JD4*MJE614;
JU24 = JD4*MJE624;
JU34 = JD4*TKT635;
JU44 = JD4*MJE644;
JU54 = JD4*MJE654;
JU64 = JD4*MJE664;
GK114 = -JU14*MJE614 + MJE114;
GK214 = -JU24*MJE614 + TKT215;
GK314 = -JU34*MJE614 + TKT315;
GK414 = -JU44*MJE614 + TKT415;
GK514 = -JU54*MJE614 + MJE514;
GK614 = -JU64*MJE614 + MJE614;
GK124 = -JU14*MJE624 + TKT215;
GK224 = -JU24*MJE624 + MJE224;
GK324 = -GX335 - JU34*MJE624;
GK424 = -JU44*MJE624 + MJE424;
GK524 = -GX535 - JU54*MJE624;
GK624 = -JU64*MJE624 + MJE624;
GK134 = -JU14*TKT635 + TKT315;
GK234 = -GX335 - JU24*TKT635;
GK334 = -JU34*TKT635 + MJE334;
GK434 = -JU44*TKT635 + MJE434;
GK534 = -JU54*TKT635 + MJE534;
GK634 = -JU64*TKT635 + TKT635;
GK144 = -JU14*MJE644 + TKT415;
GK244 = -JU24*MJE644 + MJE424;
GK344 = -JU34*MJE644 + MJE434;
GK444 = -JU44*MJE644 + MJE444;
GK544 = -JU54*MJE644 + MJE544;
GK644 = -JU64*MJE644 + MJE644;
GK154 = -JU14*MJE654 + MJE514;
GK254 = -GX535 - JU24*MJE654;
GK354 = -JU34*MJE654 + MJE534;
GK454 = -JU44*MJE654 + MJE544;
GK554 = -JU54*MJE654 + MJE554;
GK654 = -JU64*MJE654 + MJE654;
GK164 = -JU14*MJE664 + MJE614;
GK264 = -JU24*MJE664 + MJE624;
GK364 = -JU34*MJE664 + TKT635;
GK464 = -JU44*MJE664 + MJE644;
GK564 = -JU54*MJE664 + MJE654;
GK664 = -JU64*MJE664 + MJE664;
NG14 = GK144*WQ14 + GK154*WQ24;
NG24 = GK244*WQ14 + GK254*WQ24;
NG34 = GK344*WQ14 + GK354*WQ24;
NG44 = GK444*WQ14 + GK454*WQ24;
NG54 = GK544*WQ14 + GK554*WQ24;
NG64 = GK644*WQ14 + GK654*WQ24;
VS14 = GW4*JU14 + NG14;
VS24 = GW4*JU24 + NG24;
VS34 = GW4*JU34 + NG34;
VS44 = GW4*JU44 + NG44;
VS54 = GW4*JU54 + NG54;
VS64 = GW4*JU64 + NG64;
AP14 = -VBE14 + VS14;
AP24 = -VBE24 + VS24;
AP34 = -VBE34 + VS34;
AP44 = -VBE44 + VS44;
AP54 = -VBE54 + VS54;
AP64 = -VBE64 + VS64;
GX114 = C4*GK114 - GK214*S4;
GX314 = -C4*GK214 - GK114*S4;
GX414 = C4*GK414 - GK514*S4;
GX614 = -C4*GK514 - GK414*S4;
GX124 = C4*GK124 - GK224*S4;
GX324 = -C4*GK224 - GK124*S4;
GX424 = C4*GK424 - GK524*S4;
GX624 = -C4*GK524 - GK424*S4;
GX134 = C4*GK134 - GK234*S4;
GX334 = -C4*GK234 - GK134*S4;
GX434 = C4*GK434 - GK534*S4;
GX634 = -C4*GK534 - GK434*S4;
GX144 = C4*GK144 - GK244*S4;
GX344 = -C4*GK244 - GK144*S4;
GX444 = C4*GK444 - GK544*S4;
GX644 = -C4*GK544 - GK444*S4;
GX154 = C4*GK154 - GK254*S4;
GX354 = -C4*GK254 - GK154*S4;
GX454 = C4*GK454 - GK554*S4;
GX654 = -C4*GK554 - GK454*S4;
GX164 = C4*GK164 - GK264*S4;
GX364 = -C4*GK264 - GK164*S4;
GX464 = C4*GK464 - GK564*S4;
GX664 = -C4*GK564 - GK464*S4;
TKT114 = C4*GX114 - GX124*S4;
TKT214 = C4*GK314 - GK324*S4;
TKT314 = C4*GX314 - GX324*S4;
TKT414 = C4*GX414 - GX424*S4;
TKT514 = C4*GK614 - GK624*S4;
TKT614 = C4*GX614 - GX624*S4;
TKT334 = -C4*GX324 - GX314*S4;
TKT434 = -C4*GX424 - GX414*S4;
TKT534 = -C4*GK624 - GK614*S4;
TKT634 = -C4*GX624 - GX614*S4;
TKT444 = C4*GX444 - GX454*S4;
TKT544 = C4*GK644 - GK654*S4;
TKT644 = C4*GX644 - GX654*S4;
TKT664 = -C4*GX654 - GX644*S4;
ALJI14 = AP14*C4 - AP24*S4;
ALJI34 = -AP14*S4 - AP24*C4;
ALJI44 = AP44*C4 - AP54*S4;
ALJI64 = -AP44*S4 - AP54*C4;
MJE113 = M3 + TKT114;
MJE513 = MZ3 + TKT514;
MJE613 = -MY3 + TKT614;
MJE223 = GK334 + M3;
MJE423 = GX434 - MZ3;
MJE623 = GX634 + MX3;
MJE333 = M3 + TKT334;
MJE433 = MY3 + TKT434;
MJE533 = -MX3 + TKT534;
MJE443 = TKT444 + XX3;
MJE543 = TKT544 + XY3;
MJE643 = TKT644 + XZ3;
MJE553 = GK664 + YY3;
MJE653 = GX664 + YZ3;
MJE663 = TKT664 + ZZ3;
VBE13 = -ALJI14 - SW13;
VBE23 = -AP34 - SW23;
VBE33 = -ALJI34 - SW33;
VBE43 = -ALJI44 - KW13;
VBE53 = -AP64 - KW23;
VBE63 = -ALJI64 - KW33;
GW3 = GAM3 + VBE63;
JD3 = 1/MJE663;
JU13 = JD3*MJE613;
JU23 = JD3*MJE623;
JU33 = JD3*TKT634;
JU43 = JD3*MJE643;
JU53 = JD3*MJE653;
JU63 = JD3*MJE663;
GK113 = -JU13*MJE613 + MJE113;
GK213 = -JU23*MJE613 + TKT214;
GK313 = -JU33*MJE613 + TKT314;
GK413 = -JU43*MJE613 + TKT414;
GK513 = -JU53*MJE613 + MJE513;
GK613 = -JU63*MJE613 + MJE613;
GK123 = -JU13*MJE623 + TKT214;
GK223 = -JU23*MJE623 + MJE223;
GK323 = GX334 - JU33*MJE623;
GK423 = -JU43*MJE623 + MJE423;
GK523 = GK634 - JU53*MJE623;
GK623 = -JU63*MJE623 + MJE623;
GK133 = -JU13*TKT634 + TKT314;
GK233 = GX334 - JU23*TKT634;
GK333 = -JU33*TKT634 + MJE333;
GK433 = -JU43*TKT634 + MJE433;
GK533 = -JU53*TKT634 + MJE533;
GK633 = -JU63*TKT634 + TKT634;
GK143 = -JU13*MJE643 + TKT414;
GK243 = -JU23*MJE643 + MJE423;
GK343 = -JU33*MJE643 + MJE433;
GK443 = -JU43*MJE643 + MJE443;
GK543 = -JU53*MJE643 + MJE543;
GK643 = -JU63*MJE643 + MJE643;
GK153 = -JU13*MJE653 + MJE513;
GK253 = GK634 - JU23*MJE653;
GK353 = -JU33*MJE653 + MJE533;
GK453 = -JU43*MJE653 + MJE543;
GK553 = -JU53*MJE653 + MJE553;
GK653 = -JU63*MJE653 + MJE653;
GK163 = -JU13*MJE663 + MJE613;
GK263 = -JU23*MJE663 + MJE623;
GK363 = -JU33*MJE663 + TKT634;
GK463 = -JU43*MJE663 + MJE643;
GK563 = -JU53*MJE663 + MJE653;
GK663 = -JU63*MJE663 + MJE663;
NG13 = GK113*LW13 + GK123*LW23 + GK133*LW33 + GK143*WQ13 + GK153*WQ23;
NG23 = GK213*LW13 + GK223*LW23 + GK233*LW33 + GK243*WQ13 + GK253*WQ23;
NG33 = GK313*LW13 + GK323*LW23 + GK333*LW33 + GK343*WQ13 + GK353*WQ23;
NG43 = GK413*LW13 + GK423*LW23 + GK433*LW33 + GK443*WQ13 + GK453*WQ23;
NG53 = GK513*LW13 + GK523*LW23 + GK533*LW33 + GK543*WQ13 + GK553*WQ23;
NG63 = GK613*LW13 + GK623*LW23 + GK633*LW33 + GK643*WQ13 + GK653*WQ23;
VS13 = GW3*JU13 + NG13;
VS23 = GW3*JU23 + NG23;
VS33 = GW3*JU33 + NG33;
VS43 = GW3*JU43 + NG43;
VS53 = GW3*JU53 + NG53;
VS63 = GW3*JU63 + NG63;
AP13 = -VBE13 + VS13;
AP23 = -VBE23 + VS23;
AP33 = -VBE33 + VS33;
AP43 = -VBE43 + VS43;
AP53 = -VBE53 + VS53;
AP63 = -VBE63 + VS63;
GX113 = C3*GK113 - GK213*S3;
GX313 = -C3*GK213 - GK113*S3;
GX413 = C3*GK413 - GK513*S3;
GX513 = GK113*JPR123 + GK213*JPR223 + GK613;
GX613 = -C3*GK513 + 0.4*GK313 - GK413*S3;
GX123 = C3*GK123 - GK223*S3;
GX323 = -C3*GK223 - GK123*S3;
GX423 = C3*GK423 - GK523*S3;
GX523 = GK123*JPR123 + GK223*JPR223 + GK623;
GX623 = -C3*GK523 + 0.4*GK323 - GK423*S3;
GX133 = C3*GK133 - GK233*S3;
GX333 = -C3*GK233 - GK133*S3;
GX433 = C3*GK433 - GK533*S3;
GX533 = GK133*JPR123 + GK233*JPR223 + GK633;
GX633 = -C3*GK533 + 0.4*GK333 - GK433*S3;
GX143 = C3*GK143 - GK243*S3;
GX343 = -C3*GK243 - GK143*S3;
GX443 = C3*GK443 - GK543*S3;
GX543 = GK143*JPR123 + GK243*JPR223 + GK643;
GX643 = -C3*GK543 + 0.4*GK343 - GK443*S3;
GX153 = C3*GK153 - GK253*S3;
GX353 = -C3*GK253 - GK153*S3;
GX453 = C3*GK453 - GK553*S3;
GX553 = GK153*JPR123 + GK253*JPR223 + GK653;
GX653 = -C3*GK553 + 0.4*GK353 - GK453*S3;
GX163 = C3*GK163 - GK263*S3;
GX363 = -C3*GK263 - GK163*S3;
GX463 = C3*GK463 - GK563*S3;
GX563 = GK163*JPR123 + GK263*JPR223 + GK663;
GX663 = -C3*GK563 + 0.4*GK363 - GK463*S3;
TKT113 = C3*GX113 - GX123*S3;
TKT213 = C3*GK313 - GK323*S3;
TKT313 = C3*GX313 - GX323*S3;
TKT413 = C3*GX413 - GX423*S3;
TKT513 = C3*GX513 - GX523*S3;
TKT613 = C3*GX613 - GX623*S3;
TKT333 = -C3*GX323 - GX313*S3;
TKT433 = -C3*GX423 - GX413*S3;
TKT533 = -C3*GX523 - GX513*S3;
TKT633 = -C3*GX623 - GX613*S3;
TKT443 = C3*GX443 - GX453*S3;
TKT543 = C3*GX543 - GX553*S3;
TKT643 = C3*GX643 - GX653*S3;
TKT553 = GX513*JPR123 + GX523*JPR223 + GX563;
TKT653 = GX613*JPR123 + GX623*JPR223 + GX663;
TKT663 = -C3*GX653 + 0.4*GX633 - GX643*S3;
ALJI13 = AP13*C3 - AP23*S3;
ALJI33 = -AP13*S3 - AP23*C3;
ALJI43 = AP43*C3 - AP53*S3;
ALJI53 = AP13*JPR123 + AP23*JPR223 + AP63;
ALJI63 = 0.4*AP33 - AP43*S3 - AP53*C3;
MJE112 = M2 + TKT113;
MJE512 = MZ2 + TKT513;
MJE612 = -MY2 + TKT613;
MJE222 = GK333 + M2;
MJE422 = GX433 - MZ2;
MJE622 = GX633 + MX2;
MJE332 = M2 + TKT333;
MJE432 = MY2 + TKT433;
MJE532 = -MX2 + TKT533;
MJE442 = TKT443 + XX2;
MJE542 = TKT543 + XY2;
MJE642 = TKT643 + XZ2;
MJE552 = TKT553 + YY2;
MJE652 = TKT653 + YZ2;
MJE662 = TKT663 + ZZ2;
VBE12 = -ALJI13 - SW12;
VBE22 = -AP33 - SW22;
VBE32 = -ALJI33 - SW32;
VBE42 = -ALJI43 - KW12;
VBE52 = -ALJI53 - KW22;
VBE62 = -ALJI63 - KW32;
GW2 = GAM2 + VBE62;
JD2 = 1/MJE662;
JU12 = JD2*MJE612;
JU22 = JD2*MJE622;
JU32 = JD2*TKT633;
JU42 = JD2*MJE642;
JU52 = JD2*MJE652;
JU62 = JD2*MJE662;
GK112 = -JU12*MJE612 + MJE112;
GK212 = -JU22*MJE612 + TKT213;
GK312 = -JU32*MJE612 + TKT313;
GK412 = -JU42*MJE612 + TKT413;
GK512 = -JU52*MJE612 + MJE512;
GK612 = -JU62*MJE612 + MJE612;
GK122 = -JU12*MJE622 + TKT213;
GK222 = -JU22*MJE622 + MJE222;
GK322 = GX333 - JU32*MJE622;
GK422 = -JU42*MJE622 + MJE422;
GK522 = GX533 - JU52*MJE622;
GK622 = -JU62*MJE622 + MJE622;
GK132 = -JU12*TKT633 + TKT313;
GK232 = GX333 - JU22*TKT633;
GK332 = -JU32*TKT633 + MJE332;
GK432 = -JU42*TKT633 + MJE432;
GK532 = -JU52*TKT633 + MJE532;
GK632 = -JU62*TKT633 + TKT633;
GK142 = -JU12*MJE642 + TKT413;
GK242 = -JU22*MJE642 + MJE422;
GK342 = -JU32*MJE642 + MJE432;
GK442 = -JU42*MJE642 + MJE442;
GK542 = -JU52*MJE642 + MJE542;
GK642 = -JU62*MJE642 + MJE642;
GK152 = -JU12*MJE652 + MJE512;
GK252 = GX533 - JU22*MJE652;
GK352 = -JU32*MJE652 + MJE532;
GK452 = -JU42*MJE652 + MJE542;
GK552 = -JU52*MJE652 + MJE552;
GK652 = -JU62*MJE652 + MJE652;
GK162 = -JU12*MJE662 + MJE612;
GK262 = -JU22*MJE662 + MJE622;
GK362 = -JU32*MJE662 + TKT633;
GK462 = -JU42*MJE662 + MJE642;
GK562 = -JU52*MJE662 + MJE652;
GK662 = -JU62*MJE662 + MJE662;
NG12 = GK142*WQ12 + GK152*WQ22;
NG22 = GK242*WQ12 + GK252*WQ22;
NG32 = GK342*WQ12 + GK352*WQ22;
NG42 = GK442*WQ12 + GK452*WQ22;
NG52 = GK542*WQ12 + GK552*WQ22;
NG62 = GK642*WQ12 + GK652*WQ22;
VS12 = GW2*JU12 + NG12;
VS22 = GW2*JU22 + NG22;
VS32 = GW2*JU32 + NG32;
VS42 = GW2*JU42 + NG42;
VS52 = GW2*JU52 + NG52;
VS62 = GW2*JU62 + NG62;
AP12 = -VBE12 + VS12;
AP22 = -VBE22 + VS22;
AP32 = -VBE32 + VS32;
AP42 = -VBE42 + VS42;
AP52 = -VBE52 + VS52;
AP62 = -VBE62 + VS62;
GX112 = C2*GK112 - GK212*S2;
GX312 = C2*GK212 + GK112*S2;
GX412 = C2*GK412 - GK512*S2;
GX612 = C2*GK512 + GK412*S2;
GX122 = C2*GK122 - GK222*S2;
GX322 = C2*GK222 + GK122*S2;
GX422 = C2*GK422 - GK522*S2;
GX622 = C2*GK522 + GK422*S2;
GX132 = C2*GK132 - GK232*S2;
GX332 = C2*GK232 + GK132*S2;
GX432 = C2*GK432 - GK532*S2;
GX632 = C2*GK532 + GK432*S2;
GX142 = C2*GK142 - GK242*S2;
GX342 = C2*GK242 + GK142*S2;
GX442 = C2*GK442 - GK542*S2;
GX642 = C2*GK542 + GK442*S2;
GX152 = C2*GK152 - GK252*S2;
GX352 = C2*GK252 + GK152*S2;
GX452 = C2*GK452 - GK552*S2;
GX652 = C2*GK552 + GK452*S2;
GX162 = C2*GK162 - GK262*S2;
GX362 = C2*GK262 + GK162*S2;
GX462 = C2*GK462 - GK562*S2;
GX662 = C2*GK562 + GK462*S2;
TKT112 = C2*GX112 - GX122*S2;
TKT212 = -C2*GK312 + GK322*S2;
TKT312 = C2*GX312 - GX322*S2;
TKT412 = C2*GX412 - GX422*S2;
TKT512 = -C2*GK612 + GK622*S2;
TKT612 = C2*GX612 - GX622*S2;
TKT332 = C2*GX322 + GX312*S2;
TKT432 = C2*GX422 + GX412*S2;
TKT532 = -C2*GK622 - GK612*S2;
TKT632 = C2*GX622 + GX612*S2;
TKT442 = C2*GX442 - GX452*S2;
TKT542 = -C2*GK642 + GK652*S2;
TKT642 = C2*GX642 - GX652*S2;
TKT662 = C2*GX652 + GX642*S2;
ALJI12 = AP12*C2 - AP22*S2;
ALJI32 = AP12*S2 + AP22*C2;
ALJI42 = AP42*C2 - AP52*S2;
ALJI62 = AP42*S2 + AP52*C2;
MJE111 = M1 + TKT112;
MJE511 = MZ1 + TKT512;
MJE611 = -MY1 + TKT612;
MJE221 = GK332 + M1;
MJE421 = -GX432 - MZ1;
MJE621 = -GX632 + MX1;
MJE331 = M1 + TKT332;
MJE431 = MY1 + TKT432;
MJE531 = -MX1 + TKT532;
MJE441 = TKT442 + XX1;
MJE541 = TKT542 + XY1;
MJE641 = TKT642 + XZ1;
MJE551 = GK662 + YY1;
MJE651 = -GX662 + YZ1;
MJE661 = TKT662 + ZZ1;
VBE11 = -ALJI12 - SW11;
VBE21 = AP32 - SW21;
VBE41 = -ALJI42 - KW11;
VBE51 = AP62 - KW21;
GW1 = -ALJI62 + GAM1;
JD1 = 1/MJE661;
JU11 = JD1*MJE611;
JU21 = JD1*MJE621;
JU31 = JD1*TKT632;
JU41 = JD1*MJE641;
JU51 = JD1*MJE651;
JU61 = JD1*MJE661;
GK111 = -JU11*MJE611 + MJE111;
GK211 = -JU21*MJE611 + TKT212;
GK311 = -JU31*MJE611 + TKT312;
GK411 = -JU41*MJE611 + TKT412;
GK511 = -JU51*MJE611 + MJE511;
GK611 = -JU61*MJE611 + MJE611;
GK121 = -JU11*MJE621 + TKT212;
GK221 = -JU21*MJE621 + MJE221;
GK321 = -GX332 - JU31*MJE621;
GK421 = -JU41*MJE621 + MJE421;
GK521 = GK632 - JU51*MJE621;
GK621 = -JU61*MJE621 + MJE621;
GK131 = -JU11*TKT632 + TKT312;
GK231 = -GX332 - JU21*TKT632;
GK331 = -JU31*TKT632 + MJE331;
GK431 = -JU41*TKT632 + MJE431;
GK531 = -JU51*TKT632 + MJE531;
GK631 = -JU61*TKT632 + TKT632;
GK141 = -JU11*MJE641 + TKT412;
GK241 = -JU21*MJE641 + MJE421;
GK341 = -JU31*MJE641 + MJE431;
GK441 = -JU41*MJE641 + MJE441;
GK541 = -JU51*MJE641 + MJE541;
GK641 = -JU61*MJE641 + MJE641;
GK151 = -JU11*MJE651 + MJE511;
GK251 = GK632 - JU21*MJE651;
GK351 = -JU31*MJE651 + MJE531;
GK451 = -JU41*MJE651 + MJE541;
GK551 = -JU51*MJE651 + MJE551;
GK651 = -JU61*MJE651 + MJE651;
GK161 = -JU11*MJE661 + MJE611;
GK261 = -JU21*MJE661 + MJE621;
GK361 = -JU31*MJE661 + TKT632;
GK461 = -JU41*MJE661 + MJE641;
GK561 = -JU51*MJE661 + MJE651;
GK661 = -JU61*MJE661 + MJE661;
VS11 = GW1*JU11;
VS21 = GW1*JU21;
VS31 = GW1*JU31;
VS41 = GW1*JU41;
VS51 = GW1*JU51;
VS61 = GW1*JU61;
AP11 = -VBE11 + VS11;
AP21 = -VBE21 + VS21;
AP31 = ALJI32 + VS31;
AP41 = -VBE41 + VS41;
AP51 = -VBE51 + VS51;
AP61 = ALJI62 + VS61;
GX111 = C1*GK111 - GK211*S1;
GX211 = C1*GK211 + GK111*S1;
GX411 = C1*GK411 - GK511*S1;
GX511 = C1*GK511 + GK411*S1;
GX121 = C1*GK121 - GK221*S1;
GX221 = C1*GK221 + GK121*S1;
GX421 = C1*GK421 - GK521*S1;
GX521 = C1*GK521 + GK421*S1;
GX131 = C1*GK131 - GK231*S1;
GX231 = C1*GK231 + GK131*S1;
GX431 = C1*GK431 - GK531*S1;
GX531 = C1*GK531 + GK431*S1;
GX141 = C1*GK141 - GK241*S1;
GX241 = C1*GK241 + GK141*S1;
GX441 = C1*GK441 - GK541*S1;
GX541 = C1*GK541 + GK441*S1;
GX151 = C1*GK151 - GK251*S1;
GX251 = C1*GK251 + GK151*S1;
GX451 = C1*GK451 - GK551*S1;
GX551 = C1*GK551 + GK451*S1;
GX161 = C1*GK161 - GK261*S1;
GX261 = C1*GK261 + GK161*S1;
GX461 = C1*GK461 - GK561*S1;
GX561 = C1*GK561 + GK461*S1;
TKT111 = C1*GX111 - GX121*S1;
TKT211 = C1*GX211 - GX221*S1;
TKT311 = C1*GK311 - GK321*S1;
TKT411 = C1*GX411 - GX421*S1;
TKT511 = C1*GX511 - GX521*S1;
TKT611 = C1*GK611 - GK621*S1;
TKT221 = C1*GX221 + GX211*S1;
TKT321 = C1*GK321 + GK311*S1;
TKT421 = C1*GX421 + GX411*S1;
TKT521 = C1*GX521 + GX511*S1;
TKT621 = C1*GK621 + GK611*S1;
TKT441 = C1*GX441 - GX451*S1;
TKT541 = C1*GX541 - GX551*S1;
TKT641 = C1*GK641 - GK651*S1;
TKT551 = C1*GX551 + GX541*S1;
TKT651 = C1*GK651 + GK641*S1;
ALJI11 = AP11*C1 - AP21*S1;
ALJI21 = AP11*S1 + AP21*C1;
ALJI41 = AP41*C1 - AP51*S1;
ALJI51 = AP41*S1 + AP51*C1;
GU1 = -9.81*JU31;
QDP1 = -GU1 + GW1*JD1;
DY11 = MJE611*QDP1 - 9.81*TKT312;
DY21 = 9.81*GX332 + MJE621*QDP1;
DY31 = -9.81*MJE331 + QDP1*TKT632;
DY41 = -9.81*MJE431 + MJE641*QDP1;
DY51 = -9.81*MJE531 + MJE651*QDP1;
DY61 = MJE661*QDP1 - 9.81*TKT632;
E11 = DY11 - VBE11;
E21 = DY21 - VBE21;
E31 = ALJI32 + DY31;
N11 = DY41 - VBE41;
N21 = DY51 - VBE51;
N31 = ALJI62 + DY61;
VR12 = -9.81*S2;
VR22 = -9.81*C2;
VR42 = QDP1*S2 + WQ12;
VR52 = C2*QDP1 + WQ22;
GU2 = JU12*VR12 + JU22*VR22 + JU42*VR42 + JU52*VR52;
QDP2 = -GU2 + GW2*JD2;
DY12 = MJE112*VR12 + MJE512*VR52 + MJE612*QDP2 + TKT213*VR22 + TKT413*VR42;
DY22 = GX533*VR52 + MJE222*VR22 + MJE422*VR42 + MJE622*QDP2 + TKT213*VR12;
DY32 = GX333*VR22 + MJE432*VR42 + MJE532*VR52 + QDP2*TKT633 + TKT313*VR12;
DY42 = MJE422*VR22 + MJE442*VR42 + MJE542*VR52 + MJE642*QDP2 + TKT413*VR12;
DY52 = GX533*VR22 + MJE512*VR12 + MJE542*VR42 + MJE552*VR52 + MJE652*QDP2;
DY62 = MJE612*VR12 + MJE622*VR22 + MJE642*VR42 + MJE652*VR52 + MJE662*QDP2;
E12 = DY12 - VBE12;
E22 = DY22 - VBE22;
E32 = DY32 - VBE32;
N12 = DY42 - VBE42;
N22 = DY52 - VBE52;
N32 = DY62 - VBE62;
VR13 = C3*VR12 + JPR123*VR52 + LW13;
VR23 = JPR223*VR52 + LW23 - S3*VR12;
VR33 = LW33 + 0.4*QDP2 + VR22;
VR43 = C3*VR42 - QDP2*S3 + WQ13;
VR53 = -C3*QDP2 - S3*VR42 + WQ23;
GU3 = JU13*VR13 + JU23*VR23 + JU33*VR33 + JU43*VR43 + JU53*VR53 + JU63*VR52;
QDP3 = -GU3 + GW3*JD3;
WP33 = QDP3 + VR52;
DY13 = MJE113*VR13 + MJE513*VR53 + MJE613*WP33 + TKT214*VR23 + TKT314*VR33 + TKT414*VR43;
DY23 = GK634*VR53 + GX334*VR33 + MJE223*VR23 + MJE423*VR43 + MJE623*WP33 + TKT214*VR13;
DY33 = GX334*VR23 + MJE333*VR33 + MJE433*VR43 + MJE533*VR53 + TKT314*VR13 + TKT634*WP33;
DY43 = MJE423*VR23 + MJE433*VR33 + MJE443*VR43 + MJE543*VR53 + MJE643*WP33 + TKT414*VR13;
DY53 = GK634*VR23 + MJE513*VR13 + MJE533*VR33 + MJE543*VR43 + MJE553*VR53 + MJE653*WP33;
DY63 = MJE613*VR13 + MJE623*VR23 + MJE643*VR43 + MJE653*VR53 + MJE663*WP33 + TKT634*VR33;
E13 = DY13 - VBE13;
E23 = DY23 - VBE23;
E33 = DY33 - VBE33;
N13 = DY43 - VBE43;
N23 = DY53 - VBE53;
N33 = DY63 - VBE63;
VR14 = C4*VR13 - S4*VR33;
VR24 = -C4*VR33 - S4*VR13;
VR44 = C4*VR43 - S4*WP33 + WQ14;
VR54 = -C4*WP33 - S4*VR43 + WQ24;
GU4 = JU14*VR14 + JU24*VR24 + JU34*VR23 + JU44*VR44 + JU54*VR54 + JU64*VR53;
QDP4 = -GU4 + GW4*JD4;
WP34 = QDP4 + VR53;
DY14 = MJE114*VR14 + MJE514*VR54 + MJE614*WP34 + TKT215*VR24 + TKT315*VR23 + TKT415*VR44;
DY24 = -GX335*VR23 - GX535*VR54 + MJE224*VR24 + MJE424*VR44 + MJE624*WP34 + TKT215*VR14;
DY34 = -GX335*VR24 + MJE334*VR23 + MJE434*VR44 + MJE534*VR54 + TKT315*VR14 + TKT635*WP34;
DY44 = MJE424*VR24 + MJE434*VR23 + MJE444*VR44 + MJE544*VR54 + MJE644*WP34 + TKT415*VR14;
DY54 = -GX535*VR24 + MJE514*VR14 + MJE534*VR23 + MJE544*VR44 + MJE554*VR54 + MJE654*WP34;
DY64 = MJE614*VR14 + MJE624*VR24 + MJE644*VR44 + MJE654*VR54 + MJE664*WP34 + TKT635*VR23;
E14 = DY14 - VBE14;
E24 = DY24 - VBE24;
E34 = DY34 - VBE34;
N14 = DY44 - VBE44;
N24 = DY54 - VBE54;
N34 = DY64 - VBE64;
VR15 = C5*VR14 + JPR125*VR54 + LW15 + S5*VR23;
VR25 = C5*VR23 + JPR225*VR54 + LW25 - S5*VR14;
VR35 = LW35 - VR24 - 0.39*WP34;
VR45 = C5*VR44 + S5*WP34 + WQ15;
VR55 = C5*WP34 - S5*VR44 + WQ25;
GU5 = JU15*VR15 + JU25*VR25 + JU35*VR35 + JU45*VR45 + JU55*VR55 - JU65*VR54;
QDP5 = -GU5 + GW5*JD5;
WP35 = QDP5 - VR54;
DY15 = MJE115*VR15 + MJE515*VR55 + MJE615*WP35 + TKT216*VR25 + TKT316*VR35 + TKT416*VR45;
DY25 = GK636*VR55 - GX336*VR35 + MJE225*VR25 + MJE425*VR45 + MJE625*WP35 + TKT216*VR15;
DY35 = -GX336*VR25 + MJE335*VR35 + MJE435*VR45 + MJE535*VR55 + TKT316*VR15 + TKT636*WP35;
DY45 = MJE425*VR25 + MJE435*VR35 + MJE445*VR45 + MJE545*VR55 + MJE645*WP35 + TKT416*VR15;
DY55 = GK636*VR25 + MJE515*VR15 + MJE535*VR35 + MJE545*VR45 + MJE555*VR55 + MJE655*WP35;
DY65 = MJE615*VR15 + MJE625*VR25 + MJE645*VR45 + MJE655*VR55 + MJE665*WP35 + TKT636*VR35;
E15 = DY15 - VBE15;
E25 = DY25 - VBE25;
E35 = DY35 - VBE35;
N15 = DY45 - VBE45;
N25 = DY55 - VBE55;
N35 = DY65 - VBE65;
VR16 = C6*VR15 + S6*VR35;
VR26 = C6*VR35 - S6*VR15;
VR46 = C6*VR45 + S6*WP35 + WQ16;
VR56 = C6*WP35 - S6*VR45 + WQ26;
GU6 = JU16*VR16 + JU26*VR26 - JU36*VR25 + JU46*VR46 + JU56*VR56 - JU66*VR55;
QDP6 = -GU6 + GW6*JD6;
WP36 = QDP6 - VR55;
DY16 = MJE116*VR16 + MJE516*VR56 + MJE616*WP36 - TKT317*VR25 + TKT417*VR46;
DY26 = MJE226*VR26 + MJE426*VR46 + MJE626*WP36;
DY36 = -MJE336*VR25 + MJE436*VR46 + MJE536*VR56 + TKT317*VR16 + TKT637*WP36;
DY46 = MJE426*VR26 - MJE436*VR25 + MJE446*VR46 + MJE546*VR56 + MJE646*WP36 + TKT417*VR16;
DY56 = MJE516*VR16 - MJE536*VR25 + MJE546*VR46 + MJE556*VR56 + MJE656*WP36;
DY66 = MJE616*VR16 + MJE626*VR26 + MJE646*VR46 + MJE656*VR56 + MJE666*WP36 - TKT637*VR25;
E16 = DY16 - VBE16;
E26 = DY26 - VBE26;
E36 = DY36 - VBE36;
N16 = DY46 - VBE46;
N26 = DY56 - VBE56;
N36 = DY66 - VBE66;
VR17 = C7*VR16 + S7*VR25;
VR27 = C7*VR25 - S7*VR16;
VR47 = C7*VR46 - S7*WP36 + WQ17;
VR57 = -C7*WP36 - S7*VR46 + WQ27;
GU7 = JU17*VR17 + JU27*VR27 + JU47*VR47 + JU57*VR57 + JU67*VR56;
QDP7 = -GU7 + GW7*JD7;
WP37 = QDP7 + VR56;
DY17 = M7*VR17 - MY7*WP37 + MZ7*VR57;
DY27 = M7*VR27 + MX7*WP37 - MZ7*VR47;
DY37 = M7*VR26 - MX7*VR57 + MY7*VR47;
DY47 = MY7*VR26 - MZ7*VR27 + VR47*XX7 + VR57*XY7 + WP37*XZ7;
DY57 = -MX7*VR26 + MZ7*VR17 + VR47*XY7 + VR57*YY7 + WP37*YZ7;
DY67 = MX7*VR27 - MY7*VR17 + VR47*XZ7 + VR57*YZ7 + WP37*ZZ7;
E17 = -BETA17 + DY17;
E27 = -BETA27 + DY27;
E37 = -BETA37 + DY37;
N17 = -BETA47 + DY47;
N27 = -BETA57 + DY57;
N37 = -BETA67 + DY67;

ddq = [QDP1 QDP2 QDP3 QDP4 QDP5 QDP6 QDP7]';
